simulink model "complete_plant_ediff_conflict_copy_Ethan’s MacBook Pro_2022_11_12"  (R2022b)
settings: Solver=FixedStepAuto  StartTime=0.0  StopTime=300  RelTol=1e-3  EnableMultiTasking=on
model workspace (MAT data in the model file):
  A = 1.0221
  A1 : Simulink.Parameter (value not decoded)
  A2 : Simulink.Parameter (value not decoded)
  ALL_TRACK_DATA : object (value not decoded)
  Af = 1.0221
  B1 : Simulink.Parameter (value not decoded)
  B2 : Simulink.Parameter (value not decoded)
  B3 : Simulink.Parameter (value not decoded)
  BattCap = 16
  BattCap_I = 16
  C1 : Simulink.Parameter (value not decoded)
  C2 : Simulink.Parameter (value not decoded)
  C3 : Simulink.Parameter (value not decoded)
  C4 : Simulink.Parameter (value not decoded)
  C_param : Simulink.Parameter (value not decoded)
  Cd = 1.149
  FZ_C : Simulink.Parameter (value not decoded)
  Fx_limit : Simulink.Parameter (value not decoded)
  I : Simulink.Parameter (value not decoded)
  IYY_Tire = 0.3
  J_z : Simulink.Parameter (value not decoded)
  Ku : Simulink.Parameter (value not decoded)
  Motor_T_I = [30 30]
  Np = 4
  Ns = 80
  P : Simulink.Parameter (value not decoded)
  RE : Simulink.Parameter (value not decoded)
  RIM_RADIUS = 0.1524
  Rm = 0.079375
  S1 : Simulink.Parameter (value not decoded)
  S2 : Simulink.Parameter (value not decoded)
  S3 : Simulink.Parameter (value not decoded)
  S4 : Simulink.Parameter (value not decoded)
  SL_limit : Simulink.Parameter (value not decoded)
  T : Simulink.Parameter (value not decoded)
  T2F : Simulink.Parameter (value not decoded)
  Tair = 293
  V_target : Simulink.Parameter (value not decoded)
  Vg_ref = 10
  Vth : Simulink.Parameter (value not decoded)
  Vx_I = 0
  Vy_I = 0
  WHEEL_WIDTH = 0.1524
  a : Simulink.Parameter (value not decoded)
  abs_max_torque : Simulink.Parameter (value not decoded)
  absolute_battery_power_limits : Simulink.Parameter (value not decoded)
  b : Simulink.Parameter (value not decoded)
  brake_bias = [0.65 0.65 0.35 0.35]
  brakecoeff : Simulink.Parameter (value not decoded)
  c : Simulink.Parameter (value not decoded)
  cl = 2.11014
  d : Simulink.Parameter (value not decoded)
  dTx : Simulink.Parameter (value not decoded)
  dZ = 0.295
  d_bore = 0.0254
  deadband_angle : Simulink.Parameter (value not decoded)
  deadband_velocity : Simulink.Parameter (value not decoded)
  deg2rad : Simulink.Parameter (value not decoded)
  di2bp = 20
  distance_traveled = 75
  efficiency_grid : Simulink.Parameter (value not decoded)
  g : Simulink.Parameter (value not decoded)
  gr : Simulink.Parameter (value not decoded)
  inch2mm : Simulink.Parameter (value not decoded)
  k_limit : Simulink.Parameter (value not decoded)
  kx = 200
  l : Simulink.Parameter (value not decoded)
  lateral_coeff : Simulink.Parameter (value not decoded)
  m = 320
  m_tire_f = 6
  m_tire_r = 16
  max_delta_omega : Simulink.Parameter (value not decoded)
  max_motor_temp : Simulink.Parameter (value not decoded)
  max_rpm : Simulink.Parameter (value not decoded)
  max_torque : Simulink.Parameter (value not decoded)
  max_yaw_field : Simulink.Parameter (value not decoded)
  mcp_Motor = 573
  min_velocity_regen : Simulink.Parameter (value not decoded)
  motor_efficiency : Simulink.Parameter (value not decoded)
  motor_enable : Simulink.Parameter (value not decoded)
  mu_factor : Simulink.Parameter (value not decoded)
  mu_k_brake = 0.4
  mu_s_brake = 0.5
  power_input_grid : Simulink.Parameter (value not decoded)
  power_loss_grid : Simulink.Parameter (value not decoded)
  power_loss_limit : Simulink.Parameter (value not decoded)
  rho = 1.225
  rpm_index_calibration : Simulink.Parameter (value not decoded)
  rpm_sweep : Simulink.Parameter (value not decoded)
  s : Simulink.Parameter (value not decoded)
  steer_slope : Simulink.Parameter (value not decoded)
  t : Simulink.Parameter (value not decoded)
  tau : Simulink.Parameter (value not decoded)
  time_delay = 0.022
  torque_sweep : Simulink.Parameter (value not decoded)
  track_type = 1
  voltage_grid : Simulink.Parameter (value not decoded)
  yaw_I = 0
  yaw_deadband : Simulink.Parameter (value not decoded)
  yaw_error_limit : Simulink.Parameter (value not decoded)
symbols that are objects in the model workspace (value not decoded): ALL_TRACK_DATA, efficiency_grid, gr, inch2mm, l, max_rpm, max_torque, power_input_grid, RE, rpm_index_calibration, rpm_sweep, s, S1, S2, S3, S4, steer_slope, torque_sweep, voltage_grid
undefined symbols (not defined in the file): accel, ang, ang_vel, battery_voltage, brake_pressure, DiscIntNeverNeededParam, Driver, driver_input, F0z, FZ, motor_T, omega, power_limits, Reference, shock_displacement, shock_velocity, steering_angle, VEH, vel
libraries: fl_lib x20, nesl_utility x12, vehdynlibtire x10, vehdynlibsuspension x8, autolibutils x5, sharedtransform x5, sdl_lib x4, slpidlib x2, shared6dof x2, simulink x1, autolibdatasheetbattery x1, autolibmappedmotor x1
(part 10 of 10)

== system complete_plant_ediff_conflict_copy_Ethan’s MacBook Pro_2022_11_12/Vehicle Model/Wheels and Tires/VDBS/Tires/Fiala Tires/z ==
  In1 : Inport
  In2 : Inport  Port=2
  In3 : Inport  Port=3
  In4 : Inport  Port=4
  Bus Selector{,1..3} (4 alike) : BusSelector  OutputSignals=z
  Vector Concatenate : Concatenate  NumInputs=4
  Out1 : Outport  VectorParamsAs1DForOutWhenUnconnected=off
  wires:
  Bus Selector3/1 -> Vector Concatenate/4  "<z>"
  Bus Selector2/1 -> Vector Concatenate/3  "<z>"
  Bus Selector1/1 -> Vector Concatenate/2  "<z>"
  In4/1 -> Bus Selector3/1
  In3/1 -> Bus Selector2/1
  In2/1 -> Bus Selector1/1
  Bus Selector/1 -> Vector Concatenate/1  "<z>"
  In1/1 -> Bus Selector/1
  Vector Concatenate/1 -> Out1/1

== system complete_plant_ediff_conflict_copy_Ethan’s MacBook Pro_2022_11_12/Vehicle Model/Wheels and Tires/VDBS/Tires/Fiala Tires/zdot ==
  In1 : Inport
  In2 : Inport  Port=2
  In3 : Inport  Port=3
  In4 : Inport  Port=4
  Bus Selector{,1..3} (4 alike) : BusSelector  OutputSignals=zdot
  Vector Concatenate : Concatenate  NumInputs=4
  Out1 : Outport  VectorParamsAs1DForOutWhenUnconnected=off
  wires:
  Vector Concatenate/1 -> Out1/1
  In1/1 -> Bus Selector/1
  Bus Selector/1 -> Vector Concatenate/1  "<zdot>"
  In2/1 -> Bus Selector1/1
  In3/1 -> Bus Selector2/1
  In4/1 -> Bus Selector3/1
  Bus Selector1/1 -> Vector Concatenate/2  "<zdot>"
  Bus Selector2/1 -> Vector Concatenate/3  "<zdot>"
  Bus Selector3/1 -> Vector Concatenate/4  "<zdot>"

== system complete_plant_ediff_conflict_copy_Ethan’s MacBook Pro_2022_11_12/Vehicle Model/Wheels and Tires/VDBS/Tires/MF Tires/Fx ==
  In1 : Inport
  In2 : Inport  Port=2
  In3 : Inport  Port=3
  In4 : Inport  Port=4
  Bus Selector{,1..3} (4 alike) : BusSelector  OutputSignals=Fx
  Vector Concatenate : Concatenate  NumInputs=4
  Out1 : Outport  VectorParamsAs1DForOutWhenUnconnected=off
  wires:
  Bus Selector3/1 -> Vector Concatenate/4  "<Fx>"
  Bus Selector2/1 -> Vector Concatenate/3  "<Fx>"
  Bus Selector1/1 -> Vector Concatenate/2  "<Fx>"
  In4/1 -> Bus Selector3/1
  In3/1 -> Bus Selector2/1
  In2/1 -> Bus Selector1/1
  Bus Selector/1 -> Vector Concatenate/1  "<Fx>"
  In1/1 -> Bus Selector/1
  Vector Concatenate/1 -> Out1/1

== system complete_plant_ediff_conflict_copy_Ethan’s MacBook Pro_2022_11_12/Vehicle Model/Wheels and Tires/VDBS/Tires/MF Tires/Fy ==
  In1 : Inport
  In2 : Inport  Port=2
  In3 : Inport  Port=3
  In4 : Inport  Port=4
  Bus Selector{,1..3} (4 alike) : BusSelector  OutputSignals=Fy
  Vector Concatenate : Concatenate  NumInputs=4
  Out1 : Outport  VectorParamsAs1DForOutWhenUnconnected=off
  wires:
  Vector Concatenate/1 -> Out1/1
  In1/1 -> Bus Selector/1
  Bus Selector/1 -> Vector Concatenate/1  "<Fy>"
  In2/1 -> Bus Selector1/1
  In3/1 -> Bus Selector2/1
  In4/1 -> Bus Selector3/1
  Bus Selector1/1 -> Vector Concatenate/2  "<Fy>"
  Bus Selector2/1 -> Vector Concatenate/3  "<Fy>"
  Bus Selector3/1 -> Vector Concatenate/4  "<Fy>"

== system complete_plant_ediff_conflict_copy_Ethan’s MacBook Pro_2022_11_12/Vehicle Model/Wheels and Tires/VDBS/Tires/MF Tires/Fz ==
  In1 : Inport
  In2 : Inport  Port=2
  In3 : Inport  Port=3
  In4 : Inport  Port=4
  Bus Selector{,1..3} (4 alike) : BusSelector  OutputSignals=Fz
  Vector Concatenate : Concatenate  NumInputs=4
  Out1 : Outport  VectorParamsAs1DForOutWhenUnconnected=off
  wires:
  Vector Concatenate/1 -> Out1/1
  In1/1 -> Bus Selector/1
  Bus Selector/1 -> Vector Concatenate/1  "<Fz>"
  In2/1 -> Bus Selector1/1
  In3/1 -> Bus Selector2/1
  In4/1 -> Bus Selector3/1
  Bus Selector1/1 -> Vector Concatenate/2  "<Fz>"
  Bus Selector2/1 -> Vector Concatenate/3  "<Fz>"
  Bus Selector3/1 -> Vector Concatenate/4  "<Fz>"

== system complete_plant_ediff_conflict_copy_Ethan’s MacBook Pro_2022_11_12/Vehicle Model/Wheels and Tires/VDBS/Tires/MF Tires/Mx ==
  In1 : Inport
  In2 : Inport  Port=2
  In3 : Inport  Port=3
  In4 : Inport  Port=4
  Bus Selector{,1..3} (4 alike) : BusSelector  OutputSignals=Mx
  Vector Concatenate : Concatenate  NumInputs=4
  Out1 : Outport  VectorParamsAs1DForOutWhenUnconnected=off
  wires:
  Vector Concatenate/1 -> Out1/1
  In1/1 -> Bus Selector/1
  Bus Selector/1 -> Vector Concatenate/1  "<Mx>"
  In2/1 -> Bus Selector1/1
  In3/1 -> Bus Selector2/1
  In4/1 -> Bus Selector3/1
  Bus Selector1/1 -> Vector Concatenate/2  "<Mx>"
  Bus Selector2/1 -> Vector Concatenate/3  "<Mx>"
  Bus Selector3/1 -> Vector Concatenate/4  "<Mx>"

== system complete_plant_ediff_conflict_copy_Ethan’s MacBook Pro_2022_11_12/Vehicle Model/Wheels and Tires/VDBS/Tires/MF Tires/My ==
  In1 : Inport
  In2 : Inport  Port=2
  In3 : Inport  Port=3
  In4 : Inport  Port=4
  Bus Selector{,1..3} (4 alike) : BusSelector  OutputSignals=My
  Vector Concatenate : Concatenate  NumInputs=4
  Out1 : Outport  VectorParamsAs1DForOutWhenUnconnected=off
  wires:
  Bus Selector3/1 -> Vector Concatenate/4  "<My>"
  Bus Selector2/1 -> Vector Concatenate/3  "<My>"
  Bus Selector1/1 -> Vector Concatenate/2  "<My>"
  In4/1 -> Bus Selector3/1
  In3/1 -> Bus Selector2/1
  In2/1 -> Bus Selector1/1
  Bus Selector/1 -> Vector Concatenate/1  "<My>"
  In1/1 -> Bus Selector/1
  Vector Concatenate/1 -> Out1/1

== system complete_plant_ediff_conflict_copy_Ethan’s MacBook Pro_2022_11_12/Vehicle Model/Wheels and Tires/VDBS/Tires/MF Tires/Mz ==
  In1 : Inport
  In2 : Inport  Port=2
  In3 : Inport  Port=3
  In4 : Inport  Port=4
  Bus Selector{,1..3} (4 alike) : BusSelector  OutputSignals=Mz
  Vector Concatenate : Concatenate  NumInputs=4
  Out1 : Outport  VectorParamsAs1DForOutWhenUnconnected=off
  wires:
  Bus Selector3/1 -> Vector Concatenate/4  "<Mz>"
  Bus Selector2/1 -> Vector Concatenate/3  "<Mz>"
  Bus Selector1/1 -> Vector Concatenate/2  "<Mz>"
  In4/1 -> Bus Selector3/1
  In3/1 -> Bus Selector2/1
  In2/1 -> Bus Selector1/1
  Bus Selector/1 -> Vector Concatenate/1  "<Mz>"
  In1/1 -> Bus Selector/1
  Vector Concatenate/1 -> Out1/1

== system complete_plant_ediff_conflict_copy_Ethan’s MacBook Pro_2022_11_12/Vehicle Model/Wheels and Tires/VDBS/Tires/MF Tires/Re ==
  In1 : Inport
  In2 : Inport  Port=2
  In3 : Inport  Port=3
  In4 : Inport  Port=4
  Bus Selector{,1..3} (4 alike) : BusSelector  OutputSignals=Re
  Vector Concatenate : Concatenate  NumInputs=4
  Out1 : Outport  VectorParamsAs1DForOutWhenUnconnected=off
  wires:
  Vector Concatenate/1 -> Out1/1
  In1/1 -> Bus Selector/1
  Bus Selector/1 -> Vector Concatenate/1  "<Re>"
  In2/1 -> Bus Selector1/1
  In3/1 -> Bus Selector2/1
  In4/1 -> Bus Selector3/1
  Bus Selector1/1 -> Vector Concatenate/2  "<Re>"
  Bus Selector2/1 -> Vector Concatenate/3  "<Re>"
  Bus Selector3/1 -> Vector Concatenate/4  "<Re>"

== system complete_plant_ediff_conflict_copy_Ethan’s MacBook Pro_2022_11_12/Vehicle Model/Wheels and Tires/VDBS/Tires/MF Tires/alpha ==
  In1 : Inport
  In2 : Inport  Port=2
  In3 : Inport  Port=3
  In4 : Inport  Port=4
  Bus Selector{,1..3} (4 alike) : BusSelector  OutputSignals=Alpha
  Vector Concatenate : Concatenate  NumInputs=4
  Out1 : Outport  VectorParamsAs1DForOutWhenUnconnected=off
  wires:
  Vector Concatenate/1 -> Out1/1
  In1/1 -> Bus Selector/1
  Bus Selector/1 -> Vector Concatenate/1  "<Alpha>"
  In2/1 -> Bus Selector1/1
  In3/1 -> Bus Selector2/1
  In4/1 -> Bus Selector3/1
  Bus Selector1/1 -> Vector Concatenate/2  "<Alpha>"
  Bus Selector2/1 -> Vector Concatenate/3  "<Alpha>"
  Bus Selector3/1 -> Vector Concatenate/4  "<Alpha>"

== system complete_plant_ediff_conflict_copy_Ethan’s MacBook Pro_2022_11_12/Vehicle Model/Wheels and Tires/VDBS/Tires/MF Tires/kappa ==
  In1 : Inport
  In2 : Inport  Port=2
  In3 : Inport  Port=3
  In4 : Inport  Port=4
  Bus Selector{,1..3} (4 alike) : BusSelector  OutputSignals=Kappa
  Vector Concatenate : Concatenate  NumInputs=4
  Out1 : Outport  VectorParamsAs1DForOutWhenUnconnected=off
  wires:
  Bus Selector3/1 -> Vector Concatenate/4  "<Kappa>"
  Bus Selector2/1 -> Vector Concatenate/3  "<Kappa>"
  Bus Selector1/1 -> Vector Concatenate/2  "<Kappa>"
  In4/1 -> Bus Selector3/1
  In3/1 -> Bus Selector2/1
  In2/1 -> Bus Selector1/1
  Bus Selector/1 -> Vector Concatenate/1  "<Kappa>"
  In1/1 -> Bus Selector/1
  Vector Concatenate/1 -> Out1/1

== system complete_plant_ediff_conflict_copy_Ethan’s MacBook Pro_2022_11_12/Vehicle Model/Wheels and Tires/VDBS/Tires/MF Tires/omega ==
  In1 : Inport
  In2 : Inport  Port=2
  In3 : Inport  Port=3
  In4 : Inport  Port=4
  Bus Selector{,1..3} (4 alike) : BusSelector  OutputSignals=Omega
  Vector Concatenate : Concatenate  NumInputs=4
  Out1 : Outport  VectorParamsAs1DForOutWhenUnconnected=off
  wires:
  In1/1 -> Bus Selector/1
  Bus Selector/1 -> Vector Concatenate/1  "<Omega>"
  In2/1 -> Bus Selector1/1
  In3/1 -> Bus Selector2/1
  In4/1 -> Bus Selector3/1
  Bus Selector1/1 -> Vector Concatenate/2  "<Omega>"
  Bus Selector2/1 -> Vector Concatenate/3  "<Omega>"
  Bus Selector3/1 -> Vector Concatenate/4  "<Omega>"
  Vector Concatenate/1 -> Out1/1

== system complete_plant_ediff_conflict_copy_Ethan’s MacBook Pro_2022_11_12/Vehicle Model/Wheels and Tires/VDBS/Tires/MF Tires/z ==
  In1 : Inport
  In2 : Inport  Port=2
  In3 : Inport  Port=3
  In4 : Inport  Port=4
  Bus Selector{,1..3} (4 alike) : BusSelector  OutputSignals=z
  Vector Concatenate : Concatenate  NumInputs=4
  Out1 : Outport  VectorParamsAs1DForOutWhenUnconnected=off
  wires:
  Bus Selector3/1 -> Vector Concatenate/4  "<z>"
  Bus Selector2/1 -> Vector Concatenate/3  "<z>"
  Bus Selector1/1 -> Vector Concatenate/2  "<z>"
  In4/1 -> Bus Selector3/1
  In3/1 -> Bus Selector2/1
  In2/1 -> Bus Selector1/1
  Bus Selector/1 -> Vector Concatenate/1  "<z>"
  In1/1 -> Bus Selector/1
  Vector Concatenate/1 -> Out1/1

== system complete_plant_ediff_conflict_copy_Ethan’s MacBook Pro_2022_11_12/Vehicle Model/Wheels and Tires/VDBS/Tires/MF Tires/zdot ==
  In1 : Inport
  In2 : Inport  Port=2
  In3 : Inport  Port=3
  In4 : Inport  Port=4
  Bus Selector{,1..3} (4 alike) : BusSelector  OutputSignals=zdot
  Vector Concatenate : Concatenate  NumInputs=4
  Out1 : Outport  VectorParamsAs1DForOutWhenUnconnected=off
  wires:
  Vector Concatenate/1 -> Out1/1
  In1/1 -> Bus Selector/1
  Bus Selector/1 -> Vector Concatenate/1  "<zdot>"
  In2/1 -> Bus Selector1/1
  In3/1 -> Bus Selector2/1
  In4/1 -> Bus Selector3/1
  Bus Selector1/1 -> Vector Concatenate/2  "<zdot>"
  Bus Selector2/1 -> Vector Concatenate/3  "<zdot>"
  Bus Selector3/1 -> Vector Concatenate/4  "<zdot>"

== matlab function complete_plant_ediff_conflict_copy_Ethan’s MacBook Pro_2022_11_12/Vehicle Model/Powertrain/Motor and Battery/MATLAB Function ==
  data: Wxx output; Wxx input size=[1 4]; Txx input size=[1 4]; T output size=[1 4]; Pmax input; Pmin input; Vbatt input; rpm_index_calibration parameter; rpm_sweep parameter; torque_sweep parameter; max_rpm parameter; power_input_grid parameter; voltage_grid parameter; max_torque parameter; k output; P output; PL_judgement output
function [Wxx, T, k, P, PL_judgement] = MC_PL(Wxx, Txx, Pmax, Pmin, Vbatt, rpm_index_calibration, rpm_sweep, torque_sweep, max_rpm, power_input_grid, voltage_grid, max_torque)
%% Calibration Conversion
    Txx = Txx;
    %Too = Too;
    Pmax = Pmax;
    Pmin = Pmin;
    Vbatt = Vbatt;


%% Input Limiting
    Txx = min(25, max(-25, Txx));
    Wxx = min(1000, max(0.01, Wxx));
    Vbatt = min(340, max(200, Vbatt));


%% Power Limits
    if sum(Txx) == 0
        Tr = [0.25 0.25 0.25 0.25];
    else
        Tr = abs((Txx.*Wxx) ./ sum(Txx.*Wxx));
    end
    
    Pmax_MC = Pmax .* Tr;
    Pmin_MC = Pmin .* Tr;
    Pxx = sign(Txx) .* interp2(rpm_sweep, torque_sweep, power_input_grid, Wxx, abs(Txx));
    
    P = min(Pmax_MC, max(Pxx, Pmin_MC));


%% Power to Torque Conversion
    T_max = pchip(max_rpm, max_torque, Wxx);
    RPM_index = ceil(Wxx ./ rpm_index_calibration);
    PL_judgement = sum((P > Pmax_MC) | (P < Pmin_MC));
    Tavg = Txx;
    
    if PL_judgement
        power_PL_lower = power_input_grid(:, RPM_index);
        power_PL_upper = power_input_grid(:, RPM_index+1);
        [~, indexOfMin_lower] = min(abs(power_PL_lower-abs(P)));
        [~, indexOfMin_upper] = min(abs(power_PL_upper-abs(P)));
    
        Ti = torque_sweep(indexOfMin_lower);    
        dTij = Ti - torque_sweep(indexOfMin_upper);    
        Wi = (RPM_index - 1) .* rpm_index_calibration;
        dWij = (RPM_index .* rpm_index_calibration) - (Wi);
        
        Tavg = sign(P) .* (Ti - (((Wxx - Wi) .* dTij) ./ dWij));
    end
    
    T = min(T_max, max(-T_max, Tavg));


%% Torque to MC Command Conversion
    V = interp2(rpm_sweep, torque_sweep, voltage_grid, Wxx, abs(T));
    k = round(4095 .* sign(T) .* min(1, V ./ Vbatt));

end

== matlab function complete_plant_ediff_conflict_copy_Ethan’s MacBook Pro_2022_11_12/Sensors/MATLAB Function1 ==
  data: Vg input; ang_vel input; sensor_left_wheel_speed output; sensor_right_wheel_speed output; s parameter
function [sensor_left_wheel_speed, sensor_right_wheel_speed] = pre_process(Vg, ang_vel, s)
%% Constants
sensor_left_wheel_speed = Vg(1) + (ang_vel(3) * s(2));
sensor_right_wheel_speed = Vg(1) + (ang_vel(3) * -s(2));

end

== matlab function complete_plant_ediff_conflict_copy_Ethan’s MacBook Pro_2022_11_12/Vehicle Model/Suspension/Double Wishbone Suspension/Steering Adapter/Compute Anti-Ackermann ==
  data: steering_angle input size=1; steering_tires output size=[1 2]; S1 parameter; S2 parameter; S3 parameter; S4 parameter; inch2mm parameter; steer_slope parameter; deg2rad parameter
function steering_tires  = anti_ackermann(steering_angle, S1, S2, S3, S4, inch2mm, steer_slope, deg2rad)
%% Inputs
% steering_angle                  [deg]


%% Outputs
% all_steering_angles             [rad][1x3]
%     steering_angle                  
%     left_steering_angle             
%     right_steering_angle            

%% Compute
rack_displacement = steer_slope * inch2mm * steering_angle;

left_steering_angle = ((S1*(rack_displacement)^3)-(S2*(rack_displacement)^2)+(S3*rack_displacement)-S4)*deg2rad;
right_steering_angle = ((S1*(rack_displacement)^3)+(S2*(rack_displacement)^2)+(S3*rack_displacement)+S4)*deg2rad;

steering_tires = [left_steering_angle, right_steering_angle];
end

== matlab function complete_plant_ediff_conflict_copy_Ethan’s MacBook Pro_2022_11_12/Driver/Longitudinal Control/MATLAB Function ==
  data: driver_input input; brake_pressure output size=[1 4]; brake_bias parameter; di2bp parameter
function brake_pressure = fcn(driver_input, brake_bias, di2bp)
    if driver_input < 0
        brake_pressure = [1 1 1 1] .* abs(driver_input) .* di2bp .* brake_bias;
    else
        brake_pressure = [0 0 0 0];
    end

end

== matlab function complete_plant_ediff_conflict_copy_Ethan’s MacBook Pro_2022_11_12/Sensors/MATLAB Function ==
  data: driver_input input; driver_input output
function driver_input = fcn(driver_input)
if driver_input < 0.01 && driver_input > -0.01
    driver_input = 0;
end

== matlab function complete_plant_ediff_conflict_copy_Ethan’s MacBook Pro_2022_11_12/Vehicle Model/Vehicle/Variant Subsystem/6DOF/Suspension to Chasiss Transforms/Estimated Unsprung Mass Orientation ==
  data: angles output size=3; angleIn input size=3; GeomXYZ output size=3; GemoXYZIn input size=3; Ground input size=4; trackW parameter; wheelB parameter
function [angles,GeomXYZ]= three26(angleIn, GemoXYZIn, Ground,trackW, wheelB)%#codegen
coder.allowpcode('plain')
% Copyright 2018 The MathWorks, Inc.
[angles,GeomXYZ]= vdynthree2six(angleIn, GemoXYZIn, Ground,trackW, wheelB);

== matlab function complete_plant_ediff_conflict_copy_Ethan’s MacBook Pro_2022_11_12/RWD Control/MATLAB Function ==
  data: yaw input; left_wheel_speed input; right_wheel_speed input; AP input; sensor_steering_wheel_angle input; prev_Tx input; Tx output size=[1 4]; filter_yaw input; filter_yaw output
function [Tx, filter_yaw]  = e_diff_c(yaw, left_wheel_speed, right_wheel_speed, AP, sensor_steering_wheel_angle, prev_Tx, filter_yaw)
% force single instead of MATLAB default double
torque_output_left = int16(0);
torque_output_right = int16(0);
filter_yaw_s = single(filter_yaw);

TxL = int16(prev_Tx(3));
TxR = int16(prev_Tx(4));

% use pass by address to output Tx
coder.ceval("eDiff", AP, left_wheel_speed, right_wheel_speed, ...
    sensor_steering_wheel_angle, TxL, TxR, yaw, coder.ref(filter_yaw_s), coder.ref(torque_output_left), coder.ref(torque_output_right));

Tx = double([0, 0, torque_output_left, torque_output_right]);
filter_yaw = double(filter_yaw_s);

end

== matlab function complete_plant_ediff_conflict_copy_Ethan’s MacBook Pro_2022_11_12/Driver/Reference Generator/Reference Geneator ==
  data: index input; steering_angle input; index output; v_error output; Vg_ref input; d_error output; psi_error output; psi input; deg2rad parameter; Vg input size=[1 2]; yaw input; x input; y input; wind_down input; ALL_TRACK_DATA parameter; v_cog output; r_ref output; r_error_2 output; x_ref output; y_ref output; wind_down output; counter output; counter input; t parameter
function [index, v_error, d_error, psi_error, v_cog, r_ref, r_error_2, x_ref, y_ref, wind_down, counter] = ref_gen(index, steering_angle, Vg_ref, psi, deg2rad, Vg, yaw, x, y, wind_down, ALL_TRACK_DATA, counter, t)
%% Extract Data
dIndex = 50;
forward_look_straight = 5;
dx = 0.1;
forward_look_turn = 15;
selected_track = ALL_TRACK_DATA.track_data_skidpad;

Y_all = selected_track(index:index+dIndex,2);
X_all = selected_track(index:index+dIndex,3);


%% Determine Reference Point
d_error_all = sqrt((Y_all - y).^2 + (X_all - x).^2);
[min_d, min_index] = min(d_error_all);
index = index + min_index - 1;


%% Aquire Reference Values
y_ref = selected_track(index, 2);
x_ref = selected_track(index, 3);
y_ref_next = selected_track(index+5, 2);
x_ref_next = selected_track(index+5, 3);
r_ref = selected_track(index, 4);
r_straight = selected_track(index+forward_look_straight, 4);
r_turn = selected_track(index+forward_look_turn, 4);
turn_ref = selected_track(index, 5);
straight_next = selected_track(index+forward_look_straight, 5);
turn_next = selected_track(index+forward_look_turn, 5);
psi_ref = selected_track(index, 8);

%% Computations
v_cog = sqrt(sum(Vg.^2));
v_error = Vg_ref - v_cog;

% Angle Error
sign_steer = 1;

if (abs(psi - psi_ref) > pi) && (sign(psi) ~= sign(psi_ref))
    if psi < 0
        sign_steer = -1;
    end
elseif (psi > psi_ref)
    sign_steer = -1;   
end

if abs(psi_ref - psi) < pi
    psi_error = sign_steer * abs(psi_ref - psi) / deg2rad;
else
    psi_error = sign_steer * ((pi - abs(psi_ref)) + (pi - abs(psi))) / deg2rad;
end

if counter > 0
    counter = counter - 1;
elseif counter < 0
    counter = counter + 1;
elseif (turn_ref ~= turn_next) && (turn_ref ~= 0) && (turn_next ~= 0)
    num = (dx*15)/(v_cog*t);
    counter = floor((dx*15)/(v_cog*t));
    wind_down = -(steering_angle) / abs(num *30*2);
elseif (turn_ref ~= turn_next) && (turn_ref ~= 0) && (turn_next == 0)
    num = (dx*5)/(v_cog*t);
    counter = floor((dx*5)/(v_cog*t));
    wind_down = -(steering_angle) / abs(num *30*2); 
else
    wind_down = 0;
end

% Turning Radius Error
if (turn_ref ~= straight_next) || (r_ref ~= r_straight)
    turn_ref = straight_next;
    r_ref = r_straight;
elseif (turn_ref ~= turn_next) && (turn_next ~= 0) && (turn_ref ~= 0)
    turn_ref = turn_next;
    r_ref = r_turn;
end

% Distance Error
indexes = [3 3.5 4 0.5 1 1.5 2 2.5 3 3.5 4 0.5 1 1.5 2 2.5 3 3.5 4 0.5 1 1.5 2 2.5 3 3.5 4];

% Determine Vehicle Quadrant
if y > y_ref
   if (x - x_ref) > 0.05
       Qc = 5;
   elseif (x - x_ref) < -0.05
       Qc = 11;
   else
       Qc = 4;
   end
elseif y < y_ref
   if (x - x_ref) > 0.05
       Qc = 7;
   elseif (x - x_ref) < -0.05
       Qc = 9;
   else
       Qc = 8;
   end
else
   if (x - x_ref) > 0.05
       Qc = 6;
   elseif (x - x_ref) < -0.05
       Qc = 10;
   else
       Qc = 0;
   end
end

% Determine Next Reference Point Quadrant
if y_ref_next > y_ref
   if x_ref_next > x_ref
       Qn = 5;
   elseif x_ref_next < x_ref
       Qn = 11;
   else
       Qn = 4;
   end
elseif y_ref_next < y_ref
   if x_ref_next > x_ref
       Qn = 7;
   elseif x_ref_next < x_ref
       Qn = 9;
   else
       Qn = 8;
   end
else
   if x_ref_next > x_ref
       Qn = 6;
   elseif x_ref_next < x_ref
       Qn = 10;
   else
       Qn = 0;
   end
end

% Determine Sign for Distance Error
if Qc == 0
    sign_distance = 0;
elseif ((mod(Qc, 1) == 0.5) && ((Qc == Qn) || (indexes(Qc+4) == Qn)))
    sign_distance = 0;
elseif (abs(x_ref_next - x_ref) == abs(x - x_ref)) && (abs(y_ref_next - y_ref) == abs(y - y_ref))
    sign_distance = 0;
elseif ((Qc ~= Qn) && (indexes(Qc+4) ~= Qn))
    if (indexes(Qc+1) == indexes(Qn)) || (indexes(Qc+2) == indexes(Qn)) || (indexes(Qc+3) == indexes(Qn))
        sign_distance = -1;
    else
        sign_distance = 1;
    end
else
    if indexes(Qc) == 1 || indexes(Qc) == 3
        y_axis = y_ref;
    elseif indexes(Qc) == 4
        y_axis = y_ref + 1;
    else
        y_axis = y_ref - 1;
    end

    if indexes(Qc) == 2 || indexes(Qc) == 4
        x_axis = x_ref;
    elseif indexes(Qc) == 1
        x_axis = x_ref + 1;
    else
        x_axis = x_ref - 1;
    end

    axis_coordiantes = [y_axis, x_axis];
    ref_coordiantes = [y_ref, x_ref];
    next_ref_coordinates = [y_ref_next, x_ref_next];
    vehicle_coordinates = [y, x];
    
    ref_vec = axis_coordiantes - ref_coordiantes;
    veh_vec = vehicle_coordinates - ref_coordiantes;
    next_ref = next_ref_coordinates - ref_coordiantes;
    
    theta_veh_ref = acos(dot(ref_vec, veh_vec) / (norm(ref_vec)*norm(veh_vec)));
    theta_next_ref = acos(dot(ref_vec, next_ref) / (norm(ref_vec)*norm(next_ref)));

    if theta_veh_ref < theta_next_ref
        sign_distance = 1;
    else
        sign_distance = -1;
    end
end

if min_d < 0.0005 && min_d > 0
    d_error = 0.0001;
elseif min_d < 0 && min_d > -0.0005
    d_error = -0.0001;
else
    d_error = sign_distance * min_d;
end

r_IC = abs(v_cog / yaw);
r_error_2 = turn_ref *  ((1 / r_ref) - (1 / r_IC));

end
